simulink library "mylib"  (R2020a)
settings: Solver=VariableStepAuto  StartTime=0.0  StopTime=10.0  RelTol=1e-3
undefined symbols (not defined in the file): d_du_max_pu, dir_to_bus1, dir_to_bus_0L, dir_to_bus_2, dir_to_line1, dir_to_line_0L, dir_to_line_2, du_max_pu, du_ph_max_pu, Fi_0, Fi_T_H, Fi_T_L, Fi_T_M, I0_calc_0L, I0_comp_H, I0_comp_L, I0_comp_M, I0_max_0L, I2_max_2, I_diff1, I_diff2, I_diff3, I_diff4, I_diff5, I_diff_to, I_hight_CT1_G, I_hight_CT2_G, I_low_CT1, I_low_CT2, I_max1, I_max2, I_max3, I_max4, I_max5, I_min_sec_CT1, I_min_sec_CT2, I_unb, Iph_max_0L, Iph_max_2, jmp_in_zone, jmp_in_zone_0L, jmp_in_zone_2, K_dop, max_min1, only_K1_0L, only_K1_2, only_K2_0L, only_K2_2, only_K3_0L, only_K3_2, P_ctl_0, PQ_Fi_ctl_0, Q_ctl_0, S_set_0, set, set1, T_fast, T_I_ctl, T_off, T_on ... (+15)
libraries: $bdroot x184, powerlib_meascontrol x97
(part 9 of 14)

== system mylib/264_DZ_trans_st_v1/Poly12_det19_ph/Za/stp_12 ==
  Y_in : Inport
  alg_in : Inport  Port=2
  Re_cur : Inport  Port=3
  Im_cur : Inport  Port=4
  Re_next : Inport  Port=5
  Im_next : Inport  Port=6
  re : Inport  Port=7
  im : Inport  Port=8
  start_pt : Inport  Port=9
  Re_start : Inport  Port=10
  Im_start : Inport  Port=11
  Constant : Constant  Value=0
  Constant1 : Constant  Value=0
  D1 : Logic  AllPortsSameDT=off  OutDataTypeStr=boolean
  Divide : Product  Inputs=**
  Divide1 : Product  Inputs=*/
  Logical Operator1 : Logic  Inputs=3  AllPortsSameDT=off  OutDataTypeStr=boolean
  Logical Operator2 : Logic  AllPortsSameDT=off  OutDataTypeStr=boolean
  Logical Operator3 : Logic  AllPortsSameDT=off  OutDataTypeStr=boolean
  Logical Operator4 : Logic  Operator=OR  AllPortsSameDT=off  OutDataTypeStr=boolean
  Logical Operator5 : Logic  AllPortsSameDT=off  OutDataTypeStr=boolean
  Logical Operator6 : Logic  Operator=OR  AllPortsSameDT=off  OutDataTypeStr=boolean
  Logical Operator7 : Logic  Operator=NOT  AllPortsSameDT=off  OutDataTypeStr=boolean
  Logical Operator8 : Logic  Operator=NOT  AllPortsSameDT=off  OutDataTypeStr=boolean
  Relational Operator{,1..3} (4 alike) : RelationalOperator  Operator===  OutDataTypeStr=boolean  RndMeth=Simplest
  Relational Operator4 : RelationalOperator  Operator=<  OutDataTypeStr=boolean  RndMeth=Simplest
  Relational Operator5 : RelationalOperator  Operator=>  OutDataTypeStr=boolean  RndMeth=Simplest
  Relational Operator6 : RelationalOperator  Operator=<  OutDataTypeStr=boolean  RndMeth=Simplest
  Relational Operator7 : RelationalOperator  Operator=>  OutDataTypeStr=boolean  RndMeth=Simplest
  Relational Operator8 : RelationalOperator  Operator=>  OutDataTypeStr=boolean  RndMeth=Simplest
  Switch{1..6} (6 alike) : Switch  Criteria=u2 > Threshold
  X2-X1 : Sum  Inputs=+-
  Y-Y1 : Sum  Inputs=+-
  Y2-Y1 : Sum  Inputs=+-
  Y2-Y2 : Sum
  Y_out : Outport
  alg_out : Outport  Port=2
  cur_Re : Outport  Port=3
  cur_Im : Outport  Port=4
  wires:
  Constant/1 -> Relational Operator1/2, Relational Operator/2
  Relational Operator1/1 -> D1/1
  Relational Operator/1 -> D1/2
  D1/1 -> Logical Operator1/1, Switch1/2, Switch2/2
  Re_next/1 -> Switch2/3, Relational Operator1/1
  Im_next/1 -> Switch1/3, Relational Operator/1
  Constant1/1 -> Relational Operator3/2, Relational Operator2/2
  Relational Operator2/1 -> Logical Operator1/3
  Relational Operator3/1 -> Logical Operator1/2
  Relational Operator4/1 -> Logical Operator2/1
  Relational Operator5/1 -> Logical Operator2/2
  Relational Operator6/1 -> Logical Operator3/1
  Relational Operator7/1 -> Logical Operator3/2
  Logical Operator2/1 -> Logical Operator4/1
  Logical Operator3/1 -> Logical Operator4/2
  Logical Operator4/1 -> Logical Operator5/1
  Logical Operator1/1 -> Logical Operator7/1
  Logical Operator7/1 -> Logical Operator6/1
  start_pt/1 -> Logical Operator6/2
  X2-X1/1 -> Divide/2
  Divide/1 -> Divide1/1
  Y2-Y1/1 -> Divide1/2
  Y-Y1/1 -> Divide/1
  Divide1/1 -> Y2-Y2/1
  Re_cur/1 -> Relational Operator3/1, X2-X1/2, Switch5/3, Y2-Y2/2
  Im_start/1 -> Switch1/1
  Re_start/1 -> Switch2/1
  re/1 -> Relational Operator8/2
  Y2-Y2/1 -> Relational Operator8/1
  im/1 -> Relational Operator7/1, Relational Operator6/1, Relational Operator5/1, Relational Operator4/1, Y-Y1/1
  Im_cur/1 -> Y2-Y1/2, Y-Y1/2, Relational Operator2/1, Switch6/3, Relational Operator6/2, Relational Operator5/2
  Switch2/1 -> X2-X1/1, Switch5/1
  Switch1/1 -> Y2-Y1/1, Switch6/1, Relational Operator7/2, Relational Operator4/2
  Relational Operator8/1 -> Logical Operator5/2
  Logical Operator5/1 -> Switch3/2
  Logical Operator6/1 -> Switch6/2, Switch5/2, Switch4/2
  Y_in/1 -> Switch4/3
  Switch3/1 -> alg_out/1, Switch4/1
  alg_in/1 -> Logical Operator8/1, Switch3/3
  Logical Operator8/1 -> Switch3/1
  Switch4/1 -> Y_out/1
  Switch6/1 -> cur_Im/1
  Switch5/1 -> cur_Re/1

== system mylib/264_DZ_trans_st_v1/Poly12_det19_ph/Za/stp_2 ==
  Y_in : Inport
  alg_in : Inport  Port=2
  Re_cur : Inport  Port=3
  Im_cur : Inport  Port=4
  Re_next : Inport  Port=5
  Im_next : Inport  Port=6
  re : Inport  Port=7
  im : Inport  Port=8
  start_pt : Inport  Port=9
  Re_start : Inport  Port=10
  Im_start : Inport  Port=11
  Constant : Constant  Value=0
  Constant1 : Constant  Value=0
  D1 : Logic  AllPortsSameDT=off  OutDataTypeStr=boolean
  Divide : Product  Inputs=**
  Divide1 : Product  Inputs=*/
  Logical Operator1 : Logic  Inputs=3  AllPortsSameDT=off  OutDataTypeStr=boolean
  Logical Operator2 : Logic  AllPortsSameDT=off  OutDataTypeStr=boolean
  Logical Operator3 : Logic  AllPortsSameDT=off  OutDataTypeStr=boolean
  Logical Operator4 : Logic  Operator=OR  AllPortsSameDT=off  OutDataTypeStr=boolean
  Logical Operator5 : Logic  AllPortsSameDT=off  OutDataTypeStr=boolean
  Logical Operator6 : Logic  Operator=OR  AllPortsSameDT=off  OutDataTypeStr=boolean
  Logical Operator7 : Logic  Operator=NOT  AllPortsSameDT=off  OutDataTypeStr=boolean
  Logical Operator8 : Logic  Operator=NOT  AllPortsSameDT=off  OutDataTypeStr=boolean
  Relational Operator{,1..3} (4 alike) : RelationalOperator  Operator===  OutDataTypeStr=boolean  RndMeth=Simplest
  Relational Operator4 : RelationalOperator  Operator=<  OutDataTypeStr=boolean  RndMeth=Simplest
  Relational Operator5 : RelationalOperator  Operator=>  OutDataTypeStr=boolean  RndMeth=Simplest
  Relational Operator6 : RelationalOperator  Operator=<  OutDataTypeStr=boolean  RndMeth=Simplest
  Relational Operator7 : RelationalOperator  Operator=>  OutDataTypeStr=boolean  RndMeth=Simplest
  Relational Operator8 : RelationalOperator  Operator=>  OutDataTypeStr=boolean  RndMeth=Simplest
  Switch{1..6} (6 alike) : Switch  Criteria=u2 > Threshold
  X2-X1 : Sum  Inputs=+-
  Y-Y1 : Sum  Inputs=+-
  Y2-Y1 : Sum  Inputs=+-
  Y2-Y2 : Sum
  Y_out : Outport
  alg_out : Outport  Port=2
  cur_Re : Outport  Port=3
  cur_Im : Outport  Port=4
  wires:
  Constant/1 -> Relational Operator1/2, Relational Operator/2
  Relational Operator1/1 -> D1/1
  Relational Operator/1 -> D1/2
  D1/1 -> Logical Operator1/1, Switch1/2, Switch2/2
  Re_next/1 -> Switch2/3, Relational Operator1/1
  Im_next/1 -> Switch1/3, Relational Operator/1
  Constant1/1 -> Relational Operator3/2, Relational Operator2/2
  Relational Operator2/1 -> Logical Operator1/3
  Relational Operator3/1 -> Logical Operator1/2
  Relational Operator4/1 -> Logical Operator2/1
  Relational Operator5/1 -> Logical Operator2/2
  Relational Operator6/1 -> Logical Operator3/1
  Relational Operator7/1 -> Logical Operator3/2
  Logical Operator2/1 -> Logical Operator4/1
  Logical Operator3/1 -> Logical Operator4/2
  Logical Operator4/1 -> Logical Operator5/1
  Logical Operator1/1 -> Logical Operator7/1
  Logical Operator7/1 -> Logical Operator6/1
  start_pt/1 -> Logical Operator6/2
  X2-X1/1 -> Divide/2
  Divide/1 -> Divide1/1
  Y2-Y1/1 -> Divide1/2
  Y-Y1/1 -> Divide/1
  Divide1/1 -> Y2-Y2/1
  Re_cur/1 -> Relational Operator3/1, X2-X1/2, Switch5/3, Y2-Y2/2
  Im_start/1 -> Switch1/1
  Re_start/1 -> Switch2/1
  re/1 -> Relational Operator8/2
  Y2-Y2/1 -> Relational Operator8/1
  im/1 -> Relational Operator7/1, Relational Operator6/1, Relational Operator5/1, Relational Operator4/1, Y-Y1/1
  Im_cur/1 -> Y2-Y1/2, Y-Y1/2, Relational Operator2/1, Switch6/3, Relational Operator6/2, Relational Operator5/2
  Switch2/1 -> X2-X1/1, Switch5/1
  Switch1/1 -> Y2-Y1/1, Switch6/1, Relational Operator7/2, Relational Operator4/2
  Relational Operator8/1 -> Logical Operator5/2
  Logical Operator5/1 -> Switch3/2
  Logical Operator6/1 -> Switch6/2, Switch5/2, Switch4/2
  Y_in/1 -> Switch4/3
  Switch3/1 -> alg_out/1, Switch4/1
  alg_in/1 -> Logical Operator8/1, Switch3/3
  Logical Operator8/1 -> Switch3/1
  Switch4/1 -> Y_out/1
  Switch6/1 -> cur_Im/1
  Switch5/1 -> cur_Re/1

== system mylib/264_DZ_trans_st_v1/Poly12_det19_ph/Za/stp_3 ==
  Y_in : Inport
  alg_in : Inport  Port=2
  Re_cur : Inport  Port=3
  Im_cur : Inport  Port=4
  Re_next : Inport  Port=5
  Im_next : Inport  Port=6
  re : Inport  Port=7
  im : Inport  Port=8
  start_pt : Inport  Port=9
  Re_start : Inport  Port=10
  Im_start : Inport  Port=11
  Constant : Constant  Value=0
  Constant1 : Constant  Value=0
  D1 : Logic  AllPortsSameDT=off  OutDataTypeStr=boolean
  Divide : Product  Inputs=**
  Divide1 : Product  Inputs=*/
  Logical Operator1 : Logic  Inputs=3  AllPortsSameDT=off  OutDataTypeStr=boolean
  Logical Operator2 : Logic  AllPortsSameDT=off  OutDataTypeStr=boolean
  Logical Operator3 : Logic  AllPortsSameDT=off  OutDataTypeStr=boolean
  Logical Operator4 : Logic  Operator=OR  AllPortsSameDT=off  OutDataTypeStr=boolean
  Logical Operator5 : Logic  AllPortsSameDT=off  OutDataTypeStr=boolean
  Logical Operator6 : Logic  Operator=OR  AllPortsSameDT=off  OutDataTypeStr=boolean
  Logical Operator7 : Logic  Operator=NOT  AllPortsSameDT=off  OutDataTypeStr=boolean
  Logical Operator8 : Logic  Operator=NOT  AllPortsSameDT=off  OutDataTypeStr=boolean
  Relational Operator{,1..3} (4 alike) : RelationalOperator  Operator===  OutDataTypeStr=boolean  RndMeth=Simplest
  Relational Operator4 : RelationalOperator  Operator=<  OutDataTypeStr=boolean  RndMeth=Simplest
  Relational Operator5 : RelationalOperator  Operator=>  OutDataTypeStr=boolean  RndMeth=Simplest
  Relational Operator6 : RelationalOperator  Operator=<  OutDataTypeStr=boolean  RndMeth=Simplest
  Relational Operator7 : RelationalOperator  Operator=>  OutDataTypeStr=boolean  RndMeth=Simplest
  Relational Operator8 : RelationalOperator  Operator=>  OutDataTypeStr=boolean  RndMeth=Simplest
  Switch{1..6} (6 alike) : Switch  Criteria=u2 > Threshold
  X2-X1 : Sum  Inputs=+-
  Y-Y1 : Sum  Inputs=+-
  Y2-Y1 : Sum  Inputs=+-
  Y2-Y2 : Sum
  Y_out : Outport
  alg_out : Outport  Port=2
  cur_Re : Outport  Port=3
  cur_Im : Outport  Port=4
  wires:
  Constant/1 -> Relational Operator1/2, Relational Operator/2
  Relational Operator1/1 -> D1/1
  Relational Operator/1 -> D1/2
  D1/1 -> Logical Operator1/1, Switch1/2, Switch2/2
  Re_next/1 -> Switch2/3, Relational Operator1/1
  Im_next/1 -> Switch1/3, Relational Operator/1
  Constant1/1 -> Relational Operator3/2, Relational Operator2/2
  Relational Operator2/1 -> Logical Operator1/3
  Relational Operator3/1 -> Logical Operator1/2
  Relational Operator4/1 -> Logical Operator2/1
  Relational Operator5/1 -> Logical Operator2/2
  Relational Operator6/1 -> Logical Operator3/1
  Relational Operator7/1 -> Logical Operator3/2
  Logical Operator2/1 -> Logical Operator4/1
  Logical Operator3/1 -> Logical Operator4/2
  Logical Operator4/1 -> Logical Operator5/1
  Logical Operator1/1 -> Logical Operator7/1
  Logical Operator7/1 -> Logical Operator6/1
  start_pt/1 -> Logical Operator6/2
  X2-X1/1 -> Divide/2
  Divide/1 -> Divide1/1
  Y2-Y1/1 -> Divide1/2
  Y-Y1/1 -> Divide/1
  Divide1/1 -> Y2-Y2/1
  Re_cur/1 -> Relational Operator3/1, X2-X1/2, Switch5/3, Y2-Y2/2
  Im_start/1 -> Switch1/1
  Re_start/1 -> Switch2/1
  re/1 -> Relational Operator8/2
  Y2-Y2/1 -> Relational Operator8/1
  im/1 -> Relational Operator7/1, Relational Operator6/1, Relational Operator5/1, Relational Operator4/1, Y-Y1/1
  Im_cur/1 -> Y2-Y1/2, Y-Y1/2, Relational Operator2/1, Switch6/3, Relational Operator6/2, Relational Operator5/2
  Switch2/1 -> X2-X1/1, Switch5/1
  Switch1/1 -> Y2-Y1/1, Switch6/1, Relational Operator7/2, Relational Operator4/2
  Relational Operator8/1 -> Logical Operator5/2
  Logical Operator5/1 -> Switch3/2
  Logical Operator6/1 -> Switch6/2, Switch5/2, Switch4/2
  Y_in/1 -> Switch4/3
  Switch3/1 -> alg_out/1, Switch4/1
  alg_in/1 -> Logical Operator8/1, Switch3/3
  Logical Operator8/1 -> Switch3/1
  Switch4/1 -> Y_out/1
  Switch6/1 -> cur_Im/1
  Switch5/1 -> cur_Re/1

== system mylib/264_DZ_trans_st_v1/Poly12_det19_ph/Za/stp_4 ==
  Y_in : Inport
  alg_in : Inport  Port=2
  Re_cur : Inport  Port=3
  Im_cur : Inport  Port=4
  Re_next : Inport  Port=5
  Im_next : Inport  Port=6
  re : Inport  Port=7
  im : Inport  Port=8
  start_pt : Inport  Port=9
  Re_start : Inport  Port=10
  Im_start : Inport  Port=11
  Constant : Constant  Value=0
  Constant1 : Constant  Value=0
  D1 : Logic  AllPortsSameDT=off  OutDataTypeStr=boolean
  Divide : Product  Inputs=**
  Divide1 : Product  Inputs=*/
  Logical Operator1 : Logic  Inputs=3  AllPortsSameDT=off  OutDataTypeStr=boolean
  Logical Operator2 : Logic  AllPortsSameDT=off  OutDataTypeStr=boolean
  Logical Operator3 : Logic  AllPortsSameDT=off  OutDataTypeStr=boolean
  Logical Operator4 : Logic  Operator=OR  AllPortsSameDT=off  OutDataTypeStr=boolean
  Logical Operator5 : Logic  AllPortsSameDT=off  OutDataTypeStr=boolean
  Logical Operator6 : Logic  Operator=OR  AllPortsSameDT=off  OutDataTypeStr=boolean
  Logical Operator7 : Logic  Operator=NOT  AllPortsSameDT=off  OutDataTypeStr=boolean
  Logical Operator8 : Logic  Operator=NOT  AllPortsSameDT=off  OutDataTypeStr=boolean
  Relational Operator{,1..3} (4 alike) : RelationalOperator  Operator===  OutDataTypeStr=boolean  RndMeth=Simplest
  Relational Operator4 : RelationalOperator  Operator=<  OutDataTypeStr=boolean  RndMeth=Simplest
  Relational Operator5 : RelationalOperator  Operator=>  OutDataTypeStr=boolean  RndMeth=Simplest
  Relational Operator6 : RelationalOperator  Operator=<  OutDataTypeStr=boolean  RndMeth=Simplest
  Relational Operator7 : RelationalOperator  Operator=>  OutDataTypeStr=boolean  RndMeth=Simplest
  Relational Operator8 : RelationalOperator  Operator=>  OutDataTypeStr=boolean  RndMeth=Simplest
  Switch{1..6} (6 alike) : Switch  Criteria=u2 > Threshold
  X2-X1 : Sum  Inputs=+-
  Y-Y1 : Sum  Inputs=+-
  Y2-Y1 : Sum  Inputs=+-
  Y2-Y2 : Sum
  Y_out : Outport
  alg_out : Outport  Port=2
  cur_Re : Outport  Port=3
  cur_Im : Outport  Port=4
  wires:
  Constant/1 -> Relational Operator1/2, Relational Operator/2
  Relational Operator1/1 -> D1/1
  Relational Operator/1 -> D1/2
  D1/1 -> Logical Operator1/1, Switch1/2, Switch2/2
  Re_next/1 -> Switch2/3, Relational Operator1/1
  Im_next/1 -> Switch1/3, Relational Operator/1
  Constant1/1 -> Relational Operator3/2, Relational Operator2/2
  Relational Operator2/1 -> Logical Operator1/3
  Relational Operator3/1 -> Logical Operator1/2
  Relational Operator4/1 -> Logical Operator2/1
  Relational Operator5/1 -> Logical Operator2/2
  Relational Operator6/1 -> Logical Operator3/1
  Relational Operator7/1 -> Logical Operator3/2
  Logical Operator2/1 -> Logical Operator4/1
  Logical Operator3/1 -> Logical Operator4/2
  Logical Operator4/1 -> Logical Operator5/1
  Logical Operator1/1 -> Logical Operator7/1
  Logical Operator7/1 -> Logical Operator6/1
  start_pt/1 -> Logical Operator6/2
  X2-X1/1 -> Divide/2
  Divide/1 -> Divide1/1
  Y2-Y1/1 -> Divide1/2
  Y-Y1/1 -> Divide/1
  Divide1/1 -> Y2-Y2/1
  Re_cur/1 -> Relational Operator3/1, X2-X1/2, Switch5/3, Y2-Y2/2
  Im_start/1 -> Switch1/1
  Re_start/1 -> Switch2/1
  re/1 -> Relational Operator8/2
  Y2-Y2/1 -> Relational Operator8/1
  im/1 -> Relational Operator7/1, Relational Operator6/1, Relational Operator5/1, Relational Operator4/1, Y-Y1/1
  Im_cur/1 -> Y2-Y1/2, Y-Y1/2, Relational Operator2/1, Switch6/3, Relational Operator6/2, Relational Operator5/2
  Switch2/1 -> X2-X1/1, Switch5/1
  Switch1/1 -> Y2-Y1/1, Switch6/1, Relational Operator7/2, Relational Operator4/2
  Relational Operator8/1 -> Logical Operator5/2
  Logical Operator5/1 -> Switch3/2
  Logical Operator6/1 -> Switch6/2, Switch5/2, Switch4/2
  Y_in/1 -> Switch4/3
  Switch3/1 -> alg_out/1, Switch4/1
  alg_in/1 -> Logical Operator8/1, Switch3/3
  Logical Operator8/1 -> Switch3/1
  Switch4/1 -> Y_out/1
  Switch6/1 -> cur_Im/1
  Switch5/1 -> cur_Re/1

== system mylib/264_DZ_trans_st_v1/Poly12_det19_ph/Za/stp_5 ==
  Y_in : Inport
  alg_in : Inport  Port=2
  Re_cur : Inport  Port=3
  Im_cur : Inport  Port=4
  Re_next : Inport  Port=5
  Im_next : Inport  Port=6
  re : Inport  Port=7
  im : Inport  Port=8
  start_pt : Inport  Port=9
  Re_start : Inport  Port=10
  Im_start : Inport  Port=11
  Constant : Constant  Value=0
  Constant1 : Constant  Value=0
  D1 : Logic  AllPortsSameDT=off  OutDataTypeStr=boolean
  Divide : Product  Inputs=**
  Divide1 : Product  Inputs=*/
  Logical Operator1 : Logic  Inputs=3  AllPortsSameDT=off  OutDataTypeStr=boolean
  Logical Operator2 : Logic  AllPortsSameDT=off  OutDataTypeStr=boolean
  Logical Operator3 : Logic  AllPortsSameDT=off  OutDataTypeStr=boolean
  Logical Operator4 : Logic  Operator=OR  AllPortsSameDT=off  OutDataTypeStr=boolean
  Logical Operator5 : Logic  AllPortsSameDT=off  OutDataTypeStr=boolean
  Logical Operator6 : Logic  Operator=OR  AllPortsSameDT=off  OutDataTypeStr=boolean
  Logical Operator7 : Logic  Operator=NOT  AllPortsSameDT=off  OutDataTypeStr=boolean
  Logical Operator8 : Logic  Operator=NOT  AllPortsSameDT=off  OutDataTypeStr=boolean
  Relational Operator{,1..3} (4 alike) : RelationalOperator  Operator===  OutDataTypeStr=boolean  RndMeth=Simplest
  Relational Operator4 : RelationalOperator  Operator=<  OutDataTypeStr=boolean  RndMeth=Simplest
  Relational Operator5 : RelationalOperator  Operator=>  OutDataTypeStr=boolean  RndMeth=Simplest
  Relational Operator6 : RelationalOperator  Operator=<  OutDataTypeStr=boolean  RndMeth=Simplest
  Relational Operator7 : RelationalOperator  Operator=>  OutDataTypeStr=boolean  RndMeth=Simplest
  Relational Operator8 : RelationalOperator  Operator=>  OutDataTypeStr=boolean  RndMeth=Simplest
  Switch{1..6} (6 alike) : Switch  Criteria=u2 > Threshold
  X2-X1 : Sum  Inputs=+-
  Y-Y1 : Sum  Inputs=+-
  Y2-Y1 : Sum  Inputs=+-
  Y2-Y2 : Sum
  Y_out : Outport
  alg_out : Outport  Port=2
  cur_Re : Outport  Port=3
  cur_Im : Outport  Port=4
  wires:
  Constant/1 -> Relational Operator1/2, Relational Operator/2
  Relational Operator1/1 -> D1/1
  Relational Operator/1 -> D1/2
  D1/1 -> Logical Operator1/1, Switch1/2, Switch2/2
  Re_next/1 -> Switch2/3, Relational Operator1/1
  Im_next/1 -> Switch1/3, Relational Operator/1
  Constant1/1 -> Relational Operator3/2, Relational Operator2/2
  Relational Operator2/1 -> Logical Operator1/3
  Relational Operator3/1 -> Logical Operator1/2
  Relational Operator4/1 -> Logical Operator2/1
  Relational Operator5/1 -> Logical Operator2/2
  Relational Operator6/1 -> Logical Operator3/1
  Relational Operator7/1 -> Logical Operator3/2
  Logical Operator2/1 -> Logical Operator4/1
  Logical Operator3/1 -> Logical Operator4/2
  Logical Operator4/1 -> Logical Operator5/1
  Logical Operator1/1 -> Logical Operator7/1
  Logical Operator7/1 -> Logical Operator6/1
  start_pt/1 -> Logical Operator6/2
  X2-X1/1 -> Divide/2
  Divide/1 -> Divide1/1
  Y2-Y1/1 -> Divide1/2
  Y-Y1/1 -> Divide/1
  Divide1/1 -> Y2-Y2/1
  Re_cur/1 -> Relational Operator3/1, X2-X1/2, Switch5/3, Y2-Y2/2
  Im_start/1 -> Switch1/1
  Re_start/1 -> Switch2/1
  re/1 -> Relational Operator8/2
  Y2-Y2/1 -> Relational Operator8/1
  im/1 -> Relational Operator7/1, Relational Operator6/1, Relational Operator5/1, Relational Operator4/1, Y-Y1/1
  Im_cur/1 -> Y2-Y1/2, Y-Y1/2, Relational Operator2/1, Switch6/3, Relational Operator6/2, Relational Operator5/2
  Switch2/1 -> X2-X1/1, Switch5/1
  Switch1/1 -> Y2-Y1/1, Switch6/1, Relational Operator7/2, Relational Operator4/2
  Relational Operator8/1 -> Logical Operator5/2
  Logical Operator5/1 -> Switch3/2
  Logical Operator6/1 -> Switch6/2, Switch5/2, Switch4/2
  Y_in/1 -> Switch4/3
  Switch3/1 -> alg_out/1, Switch4/1
  alg_in/1 -> Logical Operator8/1, Switch3/3
  Logical Operator8/1 -> Switch3/1
  Switch4/1 -> Y_out/1
  Switch6/1 -> cur_Im/1
  Switch5/1 -> cur_Re/1

== system mylib/264_DZ_trans_st_v1/Poly12_det19_ph/Za/stp_6 ==
  Y_in : Inport
  alg_in : Inport  Port=2
  Re_cur : Inport  Port=3
  Im_cur : Inport  Port=4
  Re_next : Inport  Port=5
  Im_next : Inport  Port=6
  re : Inport  Port=7
  im : Inport  Port=8
  start_pt : Inport  Port=9
  Re_start : Inport  Port=10
  Im_start : Inport  Port=11
  Constant : Constant  Value=0
  Constant1 : Constant  Value=0
  D1 : Logic  AllPortsSameDT=off  OutDataTypeStr=boolean
  Divide : Product  Inputs=**
  Divide1 : Product  Inputs=*/
  Logical Operator1 : Logic  Inputs=3  AllPortsSameDT=off  OutDataTypeStr=boolean
  Logical Operator2 : Logic  AllPortsSameDT=off  OutDataTypeStr=boolean
  Logical Operator3 : Logic  AllPortsSameDT=off  OutDataTypeStr=boolean
  Logical Operator4 : Logic  Operator=OR  AllPortsSameDT=off  OutDataTypeStr=boolean
  Logical Operator5 : Logic  AllPortsSameDT=off  OutDataTypeStr=boolean
  Logical Operator6 : Logic  Operator=OR  AllPortsSameDT=off  OutDataTypeStr=boolean
  Logical Operator7 : Logic  Operator=NOT  AllPortsSameDT=off  OutDataTypeStr=boolean
  Logical Operator8 : Logic  Operator=NOT  AllPortsSameDT=off  OutDataTypeStr=boolean
  Relational Operator{,1..3} (4 alike) : RelationalOperator  Operator===  OutDataTypeStr=boolean  RndMeth=Simplest
  Relational Operator4 : RelationalOperator  Operator=<  OutDataTypeStr=boolean  RndMeth=Simplest
  Relational Operator5 : RelationalOperator  Operator=>  OutDataTypeStr=boolean  RndMeth=Simplest
  Relational Operator6 : RelationalOperator  Operator=<  OutDataTypeStr=boolean  RndMeth=Simplest
  Relational Operator7 : RelationalOperator  Operator=>  OutDataTypeStr=boolean  RndMeth=Simplest
  Relational Operator8 : RelationalOperator  Operator=>  OutDataTypeStr=boolean  RndMeth=Simplest
  Switch{1..6} (6 alike) : Switch  Criteria=u2 > Threshold
  X2-X1 : Sum  Inputs=+-
  Y-Y1 : Sum  Inputs=+-
  Y2-Y1 : Sum  Inputs=+-
  Y2-Y2 : Sum
  Y_out : Outport
  alg_out : Outport  Port=2
  cur_Re : Outport  Port=3
  cur_Im : Outport  Port=4
  wires:
  Constant/1 -> Relational Operator1/2, Relational Operator/2
  Relational Operator1/1 -> D1/1
  Relational Operator/1 -> D1/2
  D1/1 -> Logical Operator1/1, Switch1/2, Switch2/2
  Re_next/1 -> Switch2/3, Relational Operator1/1
  Im_next/1 -> Switch1/3, Relational Operator/1
  Constant1/1 -> Relational Operator3/2, Relational Operator2/2
  Relational Operator2/1 -> Logical Operator1/3
  Relational Operator3/1 -> Logical Operator1/2
  Relational Operator4/1 -> Logical Operator2/1
  Relational Operator5/1 -> Logical Operator2/2
  Relational Operator6/1 -> Logical Operator3/1
  Relational Operator7/1 -> Logical Operator3/2
  Logical Operator2/1 -> Logical Operator4/1
  Logical Operator3/1 -> Logical Operator4/2
  Logical Operator4/1 -> Logical Operator5/1
  Logical Operator1/1 -> Logical Operator7/1
  Logical Operator7/1 -> Logical Operator6/1
  start_pt/1 -> Logical Operator6/2
  X2-X1/1 -> Divide/2
  Divide/1 -> Divide1/1
  Y2-Y1/1 -> Divide1/2
  Y-Y1/1 -> Divide/1
  Divide1/1 -> Y2-Y2/1
  Re_cur/1 -> Relational Operator3/1, X2-X1/2, Switch5/3, Y2-Y2/2
  Im_start/1 -> Switch1/1
  Re_start/1 -> Switch2/1
  re/1 -> Relational Operator8/2
  Y2-Y2/1 -> Relational Operator8/1
  im/1 -> Relational Operator7/1, Relational Operator6/1, Relational Operator5/1, Relational Operator4/1, Y-Y1/1
  Im_cur/1 -> Y2-Y1/2, Y-Y1/2, Relational Operator2/1, Switch6/3, Relational Operator6/2, Relational Operator5/2
  Switch2/1 -> X2-X1/1, Switch5/1
  Switch1/1 -> Y2-Y1/1, Switch6/1, Relational Operator7/2, Relational Operator4/2
  Relational Operator8/1 -> Logical Operator5/2
  Logical Operator5/1 -> Switch3/2
  Logical Operator6/1 -> Switch6/2, Switch5/2, Switch4/2
  Y_in/1 -> Switch4/3
  Switch3/1 -> alg_out/1, Switch4/1
  alg_in/1 -> Logical Operator8/1, Switch3/3
  Logical Operator8/1 -> Switch3/1
  Switch4/1 -> Y_out/1
  Switch6/1 -> cur_Im/1
  Switch5/1 -> cur_Re/1

== system mylib/264_DZ_trans_st_v1/Poly12_det19_ph/Za/stp_7 ==
  Y_in : Inport
  alg_in : Inport  Port=2
  Re_cur : Inport  Port=3
  Im_cur : Inport  Port=4
  Re_next : Inport  Port=5
  Im_next : Inport  Port=6
  re : Inport  Port=7
  im : Inport  Port=8
  start_pt : Inport  Port=9
  Re_start : Inport  Port=10
  Im_start : Inport  Port=11
  Constant : Constant  Value=0
  Constant1 : Constant  Value=0
  D1 : Logic  AllPortsSameDT=off  OutDataTypeStr=boolean
  Divide : Product  Inputs=**
  Divide1 : Product  Inputs=*/
  Logical Operator1 : Logic  Inputs=3  AllPortsSameDT=off  OutDataTypeStr=boolean
  Logical Operator2 : Logic  AllPortsSameDT=off  OutDataTypeStr=boolean
  Logical Operator3 : Logic  AllPortsSameDT=off  OutDataTypeStr=boolean
  Logical Operator4 : Logic  Operator=OR  AllPortsSameDT=off  OutDataTypeStr=boolean
  Logical Operator5 : Logic  AllPortsSameDT=off  OutDataTypeStr=boolean
  Logical Operator6 : Logic  Operator=OR  AllPortsSameDT=off  OutDataTypeStr=boolean
  Logical Operator7 : Logic  Operator=NOT  AllPortsSameDT=off  OutDataTypeStr=boolean
  Logical Operator8 : Logic  Operator=NOT  AllPortsSameDT=off  OutDataTypeStr=boolean
  Relational Operator{,1..3} (4 alike) : RelationalOperator  Operator===  OutDataTypeStr=boolean  RndMeth=Simplest
  Relational Operator4 : RelationalOperator  Operator=<  OutDataTypeStr=boolean  RndMeth=Simplest
  Relational Operator5 : RelationalOperator  Operator=>  OutDataTypeStr=boolean  RndMeth=Simplest
  Relational Operator6 : RelationalOperator  Operator=<  OutDataTypeStr=boolean  RndMeth=Simplest
  Relational Operator7 : RelationalOperator  Operator=>  OutDataTypeStr=boolean  RndMeth=Simplest
  Relational Operator8 : RelationalOperator  Operator=>  OutDataTypeStr=boolean  RndMeth=Simplest
  Switch{1..6} (6 alike) : Switch  Criteria=u2 > Threshold
  X2-X1 : Sum  Inputs=+-
  Y-Y1 : Sum  Inputs=+-
  Y2-Y1 : Sum  Inputs=+-
  Y2-Y2 : Sum
  Y_out : Outport
  alg_out : Outport  Port=2
  cur_Re : Outport  Port=3
  cur_Im : Outport  Port=4
  wires:
  Constant/1 -> Relational Operator1/2, Relational Operator/2
  Relational Operator1/1 -> D1/1
  Relational Operator/1 -> D1/2
  D1/1 -> Logical Operator1/1, Switch1/2, Switch2/2
  Re_next/1 -> Switch2/3, Relational Operator1/1
  Im_next/1 -> Switch1/3, Relational Operator/1
  Constant1/1 -> Relational Operator3/2, Relational Operator2/2
  Relational Operator2/1 -> Logical Operator1/3
  Relational Operator3/1 -> Logical Operator1/2
  Relational Operator4/1 -> Logical Operator2/1
  Relational Operator5/1 -> Logical Operator2/2
  Relational Operator6/1 -> Logical Operator3/1
  Relational Operator7/1 -> Logical Operator3/2
  Logical Operator2/1 -> Logical Operator4/1
  Logical Operator3/1 -> Logical Operator4/2
  Logical Operator4/1 -> Logical Operator5/1
  Logical Operator1/1 -> Logical Operator7/1
  Logical Operator7/1 -> Logical Operator6/1
  start_pt/1 -> Logical Operator6/2
  X2-X1/1 -> Divide/2
  Divide/1 -> Divide1/1
  Y2-Y1/1 -> Divide1/2
  Y-Y1/1 -> Divide/1
  Divide1/1 -> Y2-Y2/1
  Re_cur/1 -> Relational Operator3/1, X2-X1/2, Switch5/3, Y2-Y2/2
  Im_start/1 -> Switch1/1
  Re_start/1 -> Switch2/1
  re/1 -> Relational Operator8/2
  Y2-Y2/1 -> Relational Operator8/1
  im/1 -> Relational Operator7/1, Relational Operator6/1, Relational Operator5/1, Relational Operator4/1, Y-Y1/1
  Im_cur/1 -> Y2-Y1/2, Y-Y1/2, Relational Operator2/1, Switch6/3, Relational Operator6/2, Relational Operator5/2
  Switch2/1 -> X2-X1/1, Switch5/1
  Switch1/1 -> Y2-Y1/1, Switch6/1, Relational Operator7/2, Relational Operator4/2
  Relational Operator8/1 -> Logical Operator5/2
  Logical Operator5/1 -> Switch3/2
  Logical Operator6/1 -> Switch6/2, Switch5/2, Switch4/2
  Y_in/1 -> Switch4/3
  Switch3/1 -> alg_out/1, Switch4/1
  alg_in/1 -> Logical Operator8/1, Switch3/3
  Logical Operator8/1 -> Switch3/1
  Switch4/1 -> Y_out/1
  Switch6/1 -> cur_Im/1
  Switch5/1 -> cur_Re/1

== system mylib/264_DZ_trans_st_v1/Poly12_det19_ph/Za/stp_8 ==
  Y_in : Inport
  alg_in : Inport  Port=2
  Re_cur : Inport  Port=3
  Im_cur : Inport  Port=4
  Re_next : Inport  Port=5
  Im_next : Inport  Port=6
  re : Inport  Port=7
  im : Inport  Port=8
  start_pt : Inport  Port=9
  Re_start : Inport  Port=10
  Im_start : Inport  Port=11
  Constant : Constant  Value=0
  Constant1 : Constant  Value=0
  D1 : Logic  AllPortsSameDT=off  OutDataTypeStr=boolean
  Divide : Product  Inputs=**
  Divide1 : Product  Inputs=*/
  Logical Operator1 : Logic  Inputs=3  AllPortsSameDT=off  OutDataTypeStr=boolean
  Logical Operator2 : Logic  AllPortsSameDT=off  OutDataTypeStr=boolean
  Logical Operator3 : Logic  AllPortsSameDT=off  OutDataTypeStr=boolean
  Logical Operator4 : Logic  Operator=OR  AllPortsSameDT=off  OutDataTypeStr=boolean
  Logical Operator5 : Logic  AllPortsSameDT=off  OutDataTypeStr=boolean
  Logical Operator6 : Logic  Operator=OR  AllPortsSameDT=off  OutDataTypeStr=boolean
  Logical Operator7 : Logic  Operator=NOT  AllPortsSameDT=off  OutDataTypeStr=boolean
  Logical Operator8 : Logic  Operator=NOT  AllPortsSameDT=off  OutDataTypeStr=boolean
  Relational Operator{,1..3} (4 alike) : RelationalOperator  Operator===  OutDataTypeStr=boolean  RndMeth=Simplest
  Relational Operator4 : RelationalOperator  Operator=<  OutDataTypeStr=boolean  RndMeth=Simplest
  Relational Operator5 : RelationalOperator  Operator=>  OutDataTypeStr=boolean  RndMeth=Simplest
  Relational Operator6 : RelationalOperator  Operator=<  OutDataTypeStr=boolean  RndMeth=Simplest
  Relational Operator7 : RelationalOperator  Operator=>  OutDataTypeStr=boolean  RndMeth=Simplest
  Relational Operator8 : RelationalOperator  Operator=>  OutDataTypeStr=boolean  RndMeth=Simplest
  Switch{1..6} (6 alike) : Switch  Criteria=u2 > Threshold
  X2-X1 : Sum  Inputs=+-
  Y-Y1 : Sum  Inputs=+-
  Y2-Y1 : Sum  Inputs=+-
  Y2-Y2 : Sum
  Y_out : Outport
  alg_out : Outport  Port=2
  cur_Re : Outport  Port=3
  cur_Im : Outport  Port=4
  wires:
  Constant/1 -> Relational Operator1/2, Relational Operator/2
  Relational Operator1/1 -> D1/1
  Relational Operator/1 -> D1/2
  D1/1 -> Logical Operator1/1, Switch1/2, Switch2/2
  Re_next/1 -> Switch2/3, Relational Operator1/1
  Im_next/1 -> Switch1/3, Relational Operator/1
  Constant1/1 -> Relational Operator3/2, Relational Operator2/2
  Relational Operator2/1 -> Logical Operator1/3
  Relational Operator3/1 -> Logical Operator1/2
  Relational Operator4/1 -> Logical Operator2/1
  Relational Operator5/1 -> Logical Operator2/2
  Relational Operator6/1 -> Logical Operator3/1
  Relational Operator7/1 -> Logical Operator3/2
  Logical Operator2/1 -> Logical Operator4/1
  Logical Operator3/1 -> Logical Operator4/2
  Logical Operator4/1 -> Logical Operator5/1
  Logical Operator1/1 -> Logical Operator7/1
  Logical Operator7/1 -> Logical Operator6/1
  start_pt/1 -> Logical Operator6/2
  X2-X1/1 -> Divide/2
  Divide/1 -> Divide1/1
  Y2-Y1/1 -> Divide1/2
  Y-Y1/1 -> Divide/1
  Divide1/1 -> Y2-Y2/1
  Re_cur/1 -> Relational Operator3/1, X2-X1/2, Switch5/3, Y2-Y2/2
  Im_start/1 -> Switch1/1
  Re_start/1 -> Switch2/1
  re/1 -> Relational Operator8/2
  Y2-Y2/1 -> Relational Operator8/1
  im/1 -> Relational Operator7/1, Relational Operator6/1, Relational Operator5/1, Relational Operator4/1, Y-Y1/1
  Im_cur/1 -> Y2-Y1/2, Y-Y1/2, Relational Operator2/1, Switch6/3, Relational Operator6/2, Relational Operator5/2
  Switch2/1 -> X2-X1/1, Switch5/1
  Switch1/1 -> Y2-Y1/1, Switch6/1, Relational Operator7/2, Relational Operator4/2
  Relational Operator8/1 -> Logical Operator5/2
  Logical Operator5/1 -> Switch3/2
  Logical Operator6/1 -> Switch6/2, Switch5/2, Switch4/2
  Y_in/1 -> Switch4/3
  Switch3/1 -> alg_out/1, Switch4/1
  alg_in/1 -> Logical Operator8/1, Switch3/3
  Logical Operator8/1 -> Switch3/1
  Switch4/1 -> Y_out/1
  Switch6/1 -> cur_Im/1
  Switch5/1 -> cur_Re/1

== system mylib/264_DZ_trans_st_v1/Poly12_det19_ph/Za/stp_9 ==
  Y_in : Inport
  alg_in : Inport  Port=2
  Re_cur : Inport  Port=3
  Im_cur : Inport  Port=4
  Re_next : Inport  Port=5
  Im_next : Inport  Port=6
  re : Inport  Port=7
  im : Inport  Port=8
  start_pt : Inport  Port=9
  Re_start : Inport  Port=10
  Im_start : Inport  Port=11
  Constant : Constant  Value=0
  Constant1 : Constant  Value=0
  D1 : Logic  AllPortsSameDT=off  OutDataTypeStr=boolean
  Divide : Product  Inputs=**
  Divide1 : Product  Inputs=*/
  Logical Operator1 : Logic  Inputs=3  AllPortsSameDT=off  OutDataTypeStr=boolean
  Logical Operator2 : Logic  AllPortsSameDT=off  OutDataTypeStr=boolean
  Logical Operator3 : Logic  AllPortsSameDT=off  OutDataTypeStr=boolean
  Logical Operator4 : Logic  Operator=OR  AllPortsSameDT=off  OutDataTypeStr=boolean
  Logical Operator5 : Logic  AllPortsSameDT=off  OutDataTypeStr=boolean
  Logical Operator6 : Logic  Operator=OR  AllPortsSameDT=off  OutDataTypeStr=boolean
  Logical Operator7 : Logic  Operator=NOT  AllPortsSameDT=off  OutDataTypeStr=boolean
  Logical Operator8 : Logic  Operator=NOT  AllPortsSameDT=off  OutDataTypeStr=boolean
  Relational Operator{,1..3} (4 alike) : RelationalOperator  Operator===  OutDataTypeStr=boolean  RndMeth=Simplest
  Relational Operator4 : RelationalOperator  Operator=<  OutDataTypeStr=boolean  RndMeth=Simplest
  Relational Operator5 : RelationalOperator  Operator=>  OutDataTypeStr=boolean  RndMeth=Simplest
  Relational Operator6 : RelationalOperator  Operator=<  OutDataTypeStr=boolean  RndMeth=Simplest
  Relational Operator7 : RelationalOperator  Operator=>  OutDataTypeStr=boolean  RndMeth=Simplest
  Relational Operator8 : RelationalOperator  Operator=>  OutDataTypeStr=boolean  RndMeth=Simplest
  Switch{1..6} (6 alike) : Switch  Criteria=u2 > Threshold
  X2-X1 : Sum  Inputs=+-
  Y-Y1 : Sum  Inputs=+-
  Y2-Y1 : Sum  Inputs=+-
  Y2-Y2 : Sum
  Y_out : Outport
  alg_out : Outport  Port=2
  cur_Re : Outport  Port=3
  cur_Im : Outport  Port=4
  wires:
  Constant/1 -> Relational Operator1/2, Relational Operator/2
  Relational Operator1/1 -> D1/1
  Relational Operator/1 -> D1/2
  D1/1 -> Logical Operator1/1, Switch1/2, Switch2/2
  Re_next/1 -> Switch2/3, Relational Operator1/1
  Im_next/1 -> Switch1/3, Relational Operator/1
  Constant1/1 -> Relational Operator3/2, Relational Operator2/2
  Relational Operator2/1 -> Logical Operator1/3
  Relational Operator3/1 -> Logical Operator1/2
  Relational Operator4/1 -> Logical Operator2/1
  Relational Operator5/1 -> Logical Operator2/2
  Relational Operator6/1 -> Logical Operator3/1
  Relational Operator7/1 -> Logical Operator3/2
  Logical Operator2/1 -> Logical Operator4/1
  Logical Operator3/1 -> Logical Operator4/2
  Logical Operator4/1 -> Logical Operator5/1
  Logical Operator1/1 -> Logical Operator7/1
  Logical Operator7/1 -> Logical Operator6/1
  start_pt/1 -> Logical Operator6/2
  X2-X1/1 -> Divide/2
  Divide/1 -> Divide1/1
  Y2-Y1/1 -> Divide1/2
  Y-Y1/1 -> Divide/1
  Divide1/1 -> Y2-Y2/1
  Re_cur/1 -> Relational Operator3/1, X2-X1/2, Switch5/3, Y2-Y2/2
  Im_start/1 -> Switch1/1
  Re_start/1 -> Switch2/1
  re/1 -> Relational Operator8/2
  Y2-Y2/1 -> Relational Operator8/1
  im/1 -> Relational Operator7/1, Relational Operator6/1, Relational Operator5/1, Relational Operator4/1, Y-Y1/1
  Im_cur/1 -> Y2-Y1/2, Y-Y1/2, Relational Operator2/1, Switch6/3, Relational Operator6/2, Relational Operator5/2
  Switch2/1 -> X2-X1/1, Switch5/1
  Switch1/1 -> Y2-Y1/1, Switch6/1, Relational Operator7/2, Relational Operator4/2
  Relational Operator8/1 -> Logical Operator5/2
  Logical Operator5/1 -> Switch3/2
  Logical Operator6/1 -> Switch6/2, Switch5/2, Switch4/2
  Y_in/1 -> Switch4/3
  Switch3/1 -> alg_out/1, Switch4/1
  alg_in/1 -> Logical Operator8/1, Switch3/3
  Logical Operator8/1 -> Switch3/1
  Switch4/1 -> Y_out/1
  Switch6/1 -> cur_Im/1
  Switch5/1 -> cur_Re/1

== system mylib/264_DZ_trans_st_v1/Poly12_det19_ph/Zb/stp_1 ==
  Y_in : Inport
  alg_in : Inport  Port=2
  Re_cur : Inport  Port=3
  Im_cur : Inport  Port=4
  Re_next : Inport  Port=5
  Im_next : Inport  Port=6
  re : Inport  Port=7
  im : Inport  Port=8
  start_pt : Inport  Port=9
  Re_start : Inport  Port=10
  Im_start : Inport  Port=11
  Constant : Constant  Value=0
  Constant1 : Constant  Value=0
  D1 : Logic  AllPortsSameDT=off  OutDataTypeStr=boolean
  Divide : Product  Inputs=**
  Divide1 : Product  Inputs=*/
  Logical Operator1 : Logic  Inputs=3  AllPortsSameDT=off  OutDataTypeStr=boolean
  Logical Operator2 : Logic  AllPortsSameDT=off  OutDataTypeStr=boolean
  Logical Operator3 : Logic  AllPortsSameDT=off  OutDataTypeStr=boolean
  Logical Operator4 : Logic  Operator=OR  AllPortsSameDT=off  OutDataTypeStr=boolean
  Logical Operator5 : Logic  AllPortsSameDT=off  OutDataTypeStr=boolean
  Logical Operator6 : Logic  Operator=OR  AllPortsSameDT=off  OutDataTypeStr=boolean
  Logical Operator7 : Logic  Operator=NOT  AllPortsSameDT=off  OutDataTypeStr=boolean
  Logical Operator8 : Logic  Operator=NOT  AllPortsSameDT=off  OutDataTypeStr=boolean
  Relational Operator{,1..3} (4 alike) : RelationalOperator  Operator===  OutDataTypeStr=boolean  RndMeth=Simplest
  Relational Operator4 : RelationalOperator  Operator=<  OutDataTypeStr=boolean  RndMeth=Simplest
  Relational Operator5 : RelationalOperator  Operator=>  OutDataTypeStr=boolean  RndMeth=Simplest
  Relational Operator6 : RelationalOperator  Operator=<  OutDataTypeStr=boolean  RndMeth=Simplest
  Relational Operator7 : RelationalOperator  Operator=>  OutDataTypeStr=boolean  RndMeth=Simplest
  Relational Operator8 : RelationalOperator  Operator=>  OutDataTypeStr=boolean  RndMeth=Simplest
  Switch{1..6} (6 alike) : Switch  Criteria=u2 > Threshold
  X2-X1 : Sum  Inputs=+-
  Y-Y1 : Sum  Inputs=+-
  Y2-Y1 : Sum  Inputs=+-
  Y2-Y2 : Sum
  Y_out : Outport
  alg_out : Outport  Port=2
  cur_Re : Outport  Port=3
  cur_Im : Outport  Port=4
  wires:
  Constant/1 -> Relational Operator1/2, Relational Operator/2
  Relational Operator1/1 -> D1/1
  Relational Operator/1 -> D1/2
  D1/1 -> Logical Operator1/1, Switch1/2, Switch2/2
  Re_next/1 -> Switch2/3, Relational Operator1/1
  Im_next/1 -> Switch1/3, Relational Operator/1
  Constant1/1 -> Relational Operator3/2, Relational Operator2/2
  Relational Operator2/1 -> Logical Operator1/3
  Relational Operator3/1 -> Logical Operator1/2
  Relational Operator4/1 -> Logical Operator2/1
  Relational Operator5/1 -> Logical Operator2/2
  Relational Operator6/1 -> Logical Operator3/1
  Relational Operator7/1 -> Logical Operator3/2
  Logical Operator2/1 -> Logical Operator4/1
  Logical Operator3/1 -> Logical Operator4/2
  Logical Operator4/1 -> Logical Operator5/1
  Logical Operator1/1 -> Logical Operator7/1
  Logical Operator7/1 -> Logical Operator6/1
  start_pt/1 -> Logical Operator6/2
  X2-X1/1 -> Divide/2
  Divide/1 -> Divide1/1
  Y2-Y1/1 -> Divide1/2
  Y-Y1/1 -> Divide/1
  Divide1/1 -> Y2-Y2/1
  Re_cur/1 -> Relational Operator3/1, X2-X1/2, Switch5/3, Y2-Y2/2
  Im_start/1 -> Switch1/1
  Re_start/1 -> Switch2/1
  re/1 -> Relational Operator8/2
  Y2-Y2/1 -> Relational Operator8/1
  im/1 -> Relational Operator7/1, Relational Operator6/1, Relational Operator5/1, Relational Operator4/1, Y-Y1/1
  Im_cur/1 -> Y2-Y1/2, Y-Y1/2, Relational Operator2/1, Switch6/3, Relational Operator6/2, Relational Operator5/2
  Switch2/1 -> X2-X1/1, Switch5/1
  Switch1/1 -> Y2-Y1/1, Switch6/1, Relational Operator7/2, Relational Operator4/2
  Relational Operator8/1 -> Logical Operator5/2
  Logical Operator5/1 -> Switch3/2
  Logical Operator6/1 -> Switch6/2, Switch5/2, Switch4/2
  Y_in/1 -> Switch4/3
  Switch3/1 -> alg_out/1, Switch4/1
  alg_in/1 -> Logical Operator8/1, Switch3/3
  Logical Operator8/1 -> Switch3/1
  Switch4/1 -> Y_out/1
  Switch6/1 -> cur_Im/1
  Switch5/1 -> cur_Re/1

== system mylib/264_DZ_trans_st_v1/Poly12_det19_ph/Zb/stp_10 ==
  Y_in : Inport
  alg_in : Inport  Port=2
  Re_cur : Inport  Port=3
  Im_cur : Inport  Port=4
  Re_next : Inport  Port=5
  Im_next : Inport  Port=6
  re : Inport  Port=7
  im : Inport  Port=8
  start_pt : Inport  Port=9
  Re_start : Inport  Port=10
  Im_start : Inport  Port=11
  Constant : Constant  Value=0
  Constant1 : Constant  Value=0
  D1 : Logic  AllPortsSameDT=off  OutDataTypeStr=boolean
  Divide : Product  Inputs=**
  Divide1 : Product  Inputs=*/
  Logical Operator1 : Logic  Inputs=3  AllPortsSameDT=off  OutDataTypeStr=boolean
  Logical Operator2 : Logic  AllPortsSameDT=off  OutDataTypeStr=boolean
  Logical Operator3 : Logic  AllPortsSameDT=off  OutDataTypeStr=boolean
  Logical Operator4 : Logic  Operator=OR  AllPortsSameDT=off  OutDataTypeStr=boolean
  Logical Operator5 : Logic  AllPortsSameDT=off  OutDataTypeStr=boolean
  Logical Operator6 : Logic  Operator=OR  AllPortsSameDT=off  OutDataTypeStr=boolean
  Logical Operator7 : Logic  Operator=NOT  AllPortsSameDT=off  OutDataTypeStr=boolean
  Logical Operator8 : Logic  Operator=NOT  AllPortsSameDT=off  OutDataTypeStr=boolean
  Relational Operator{,1..3} (4 alike) : RelationalOperator  Operator===  OutDataTypeStr=boolean  RndMeth=Simplest
  Relational Operator4 : RelationalOperator  Operator=<  OutDataTypeStr=boolean  RndMeth=Simplest
  Relational Operator5 : RelationalOperator  Operator=>  OutDataTypeStr=boolean  RndMeth=Simplest
  Relational Operator6 : RelationalOperator  Operator=<  OutDataTypeStr=boolean  RndMeth=Simplest
  Relational Operator7 : RelationalOperator  Operator=>  OutDataTypeStr=boolean  RndMeth=Simplest
  Relational Operator8 : RelationalOperator  Operator=>  OutDataTypeStr=boolean  RndMeth=Simplest
  Switch{1..6} (6 alike) : Switch  Criteria=u2 > Threshold
  X2-X1 : Sum  Inputs=+-
  Y-Y1 : Sum  Inputs=+-
  Y2-Y1 : Sum  Inputs=+-
  Y2-Y2 : Sum
  Y_out : Outport
  alg_out : Outport  Port=2
  cur_Re : Outport  Port=3
  cur_Im : Outport  Port=4
  wires:
  Constant/1 -> Relational Operator1/2, Relational Operator/2
  Relational Operator1/1 -> D1/1
  Relational Operator/1 -> D1/2
  D1/1 -> Logical Operator1/1, Switch1/2, Switch2/2
  Re_next/1 -> Switch2/3, Relational Operator1/1
  Im_next/1 -> Switch1/3, Relational Operator/1
  Constant1/1 -> Relational Operator3/2, Relational Operator2/2
  Relational Operator2/1 -> Logical Operator1/3
  Relational Operator3/1 -> Logical Operator1/2
  Relational Operator4/1 -> Logical Operator2/1
  Relational Operator5/1 -> Logical Operator2/2
  Relational Operator6/1 -> Logical Operator3/1
  Relational Operator7/1 -> Logical Operator3/2
  Logical Operator2/1 -> Logical Operator4/1
  Logical Operator3/1 -> Logical Operator4/2
  Logical Operator4/1 -> Logical Operator5/1
  Logical Operator1/1 -> Logical Operator7/1
  Logical Operator7/1 -> Logical Operator6/1
  start_pt/1 -> Logical Operator6/2
  X2-X1/1 -> Divide/2
  Divide/1 -> Divide1/1
  Y2-Y1/1 -> Divide1/2
  Y-Y1/1 -> Divide/1
  Divide1/1 -> Y2-Y2/1
  Re_cur/1 -> Relational Operator3/1, X2-X1/2, Switch5/3, Y2-Y2/2
  Im_start/1 -> Switch1/1
  Re_start/1 -> Switch2/1
  re/1 -> Relational Operator8/2
  Y2-Y2/1 -> Relational Operator8/1
  im/1 -> Relational Operator7/1, Relational Operator6/1, Relational Operator5/1, Relational Operator4/1, Y-Y1/1
  Im_cur/1 -> Y2-Y1/2, Y-Y1/2, Relational Operator2/1, Switch6/3, Relational Operator6/2, Relational Operator5/2
  Switch2/1 -> X2-X1/1, Switch5/1
  Switch1/1 -> Y2-Y1/1, Switch6/1, Relational Operator7/2, Relational Operator4/2
  Relational Operator8/1 -> Logical Operator5/2
  Logical Operator5/1 -> Switch3/2
  Logical Operator6/1 -> Switch6/2, Switch5/2, Switch4/2
  Y_in/1 -> Switch4/3
  Switch3/1 -> alg_out/1, Switch4/1
  alg_in/1 -> Logical Operator8/1, Switch3/3
  Logical Operator8/1 -> Switch3/1
  Switch4/1 -> Y_out/1
  Switch6/1 -> cur_Im/1
  Switch5/1 -> cur_Re/1

== system mylib/264_DZ_trans_st_v1/Poly12_det19_ph/Zb/stp_11 ==
  Y_in : Inport
  alg_in : Inport  Port=2
  Re_cur : Inport  Port=3
  Im_cur : Inport  Port=4
  Re_next : Inport  Port=5
  Im_next : Inport  Port=6
  re : Inport  Port=7
  im : Inport  Port=8
  start_pt : Inport  Port=9
  Re_start : Inport  Port=10
  Im_start : Inport  Port=11
  Constant : Constant  Value=0
  Constant1 : Constant  Value=0
  D1 : Logic  AllPortsSameDT=off  OutDataTypeStr=boolean
  Divide : Product  Inputs=**
  Divide1 : Product  Inputs=*/
  Logical Operator1 : Logic  Inputs=3  AllPortsSameDT=off  OutDataTypeStr=boolean
  Logical Operator2 : Logic  AllPortsSameDT=off  OutDataTypeStr=boolean
  Logical Operator3 : Logic  AllPortsSameDT=off  OutDataTypeStr=boolean
  Logical Operator4 : Logic  Operator=OR  AllPortsSameDT=off  OutDataTypeStr=boolean
  Logical Operator5 : Logic  AllPortsSameDT=off  OutDataTypeStr=boolean
  Logical Operator6 : Logic  Operator=OR  AllPortsSameDT=off  OutDataTypeStr=boolean
  Logical Operator7 : Logic  Operator=NOT  AllPortsSameDT=off  OutDataTypeStr=boolean
  Logical Operator8 : Logic  Operator=NOT  AllPortsSameDT=off  OutDataTypeStr=boolean
  Relational Operator{,1..3} (4 alike) : RelationalOperator  Operator===  OutDataTypeStr=boolean  RndMeth=Simplest
  Relational Operator4 : RelationalOperator  Operator=<  OutDataTypeStr=boolean  RndMeth=Simplest
  Relational Operator5 : RelationalOperator  Operator=>  OutDataTypeStr=boolean  RndMeth=Simplest
  Relational Operator6 : RelationalOperator  Operator=<  OutDataTypeStr=boolean  RndMeth=Simplest
  Relational Operator7 : RelationalOperator  Operator=>  OutDataTypeStr=boolean  RndMeth=Simplest
  Relational Operator8 : RelationalOperator  Operator=>  OutDataTypeStr=boolean  RndMeth=Simplest
  Switch{1..6} (6 alike) : Switch  Criteria=u2 > Threshold
  X2-X1 : Sum  Inputs=+-
  Y-Y1 : Sum  Inputs=+-
  Y2-Y1 : Sum  Inputs=+-
  Y2-Y2 : Sum
  Y_out : Outport
  alg_out : Outport  Port=2
  cur_Re : Outport  Port=3
  cur_Im : Outport  Port=4
  wires:
  Constant/1 -> Relational Operator1/2, Relational Operator/2
  Relational Operator1/1 -> D1/1
  Relational Operator/1 -> D1/2
  D1/1 -> Logical Operator1/1, Switch1/2, Switch2/2
  Re_next/1 -> Switch2/3, Relational Operator1/1
  Im_next/1 -> Switch1/3, Relational Operator/1
  Constant1/1 -> Relational Operator3/2, Relational Operator2/2
  Relational Operator2/1 -> Logical Operator1/3
  Relational Operator3/1 -> Logical Operator1/2
  Relational Operator4/1 -> Logical Operator2/1
  Relational Operator5/1 -> Logical Operator2/2
  Relational Operator6/1 -> Logical Operator3/1
  Relational Operator7/1 -> Logical Operator3/2
  Logical Operator2/1 -> Logical Operator4/1
  Logical Operator3/1 -> Logical Operator4/2
  Logical Operator4/1 -> Logical Operator5/1
  Logical Operator1/1 -> Logical Operator7/1
  Logical Operator7/1 -> Logical Operator6/1
  start_pt/1 -> Logical Operator6/2
  X2-X1/1 -> Divide/2
  Divide/1 -> Divide1/1
  Y2-Y1/1 -> Divide1/2
  Y-Y1/1 -> Divide/1
  Divide1/1 -> Y2-Y2/1
  Re_cur/1 -> Relational Operator3/1, X2-X1/2, Switch5/3, Y2-Y2/2
  Im_start/1 -> Switch1/1
  Re_start/1 -> Switch2/1
  re/1 -> Relational Operator8/2
  Y2-Y2/1 -> Relational Operator8/1
  im/1 -> Relational Operator7/1, Relational Operator6/1, Relational Operator5/1, Relational Operator4/1, Y-Y1/1
  Im_cur/1 -> Y2-Y1/2, Y-Y1/2, Relational Operator2/1, Switch6/3, Relational Operator6/2, Relational Operator5/2
  Switch2/1 -> X2-X1/1, Switch5/1
  Switch1/1 -> Y2-Y1/1, Switch6/1, Relational Operator7/2, Relational Operator4/2
  Relational Operator8/1 -> Logical Operator5/2
  Logical Operator5/1 -> Switch3/2
  Logical Operator6/1 -> Switch6/2, Switch5/2, Switch4/2
  Y_in/1 -> Switch4/3
  Switch3/1 -> alg_out/1, Switch4/1
  alg_in/1 -> Logical Operator8/1, Switch3/3
  Logical Operator8/1 -> Switch3/1
  Switch4/1 -> Y_out/1
  Switch6/1 -> cur_Im/1
  Switch5/1 -> cur_Re/1
